simulink model "Sterowanie_StatkiemVIDI_2015"  (R2015b)
settings: Solver=FixedStepAuto  SolverMode=SingleTasking  StartTime=0.0  StopTime=10  FixedStep=0.001  MaxStep=0.01  MinStep=.009  RelTol=1e-2
settings Model: Creator=szymo  LastModifiedBy=szymo
settings SolverCC: AlgebraicLoopSolver=LineSearch
settings DataIOCC: LimitDataPoints=off  ReturnWorkspaceOutputs=on
settings DebuggingCC: AllowSymbolicDim=on  SFUnexpectedBacktrackingDiag=error  SFNoUnconditionalDefaultTransitionDiag=error
settings ModelReferenceCC: PropagateSignalLabelsOutOfModel=on
settings SFSimCC: SimUseLocalCustomCode=on
settings RTWCC: RTWUseLocalCustomCode=on
settings GRTTargetCC: TargetLangStandard=C99 (ISO)
settings ConfigComp: CovMetricSettings=dwe  CovHtmlReporting=off  CovSaveCumulativeToWorkspaceVar=off  CovSaveSingleToWorkspaceVar=off  CovModelRefEnable=Off  CovExternalEMLEnable=on

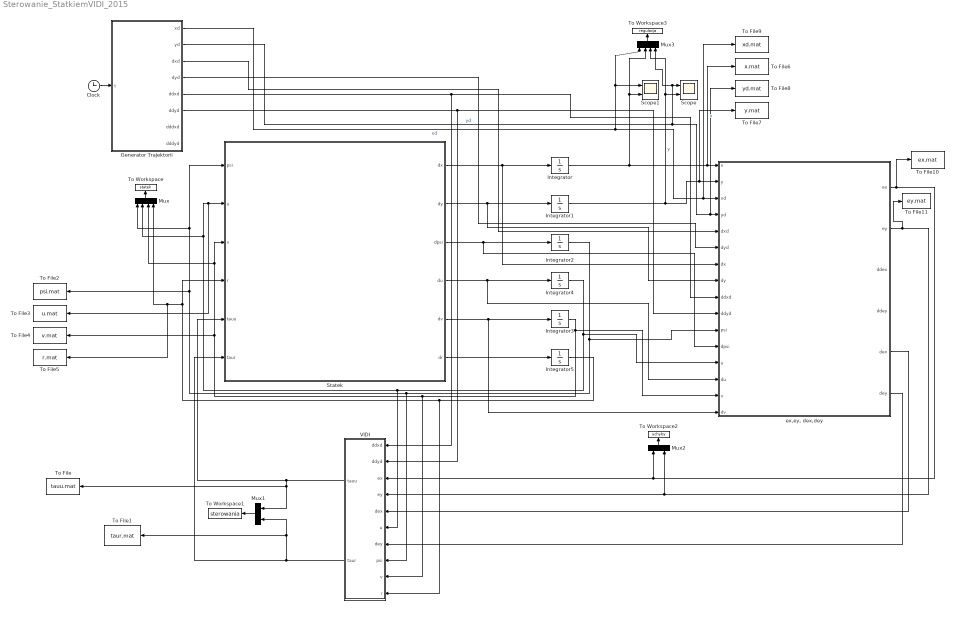
== system Sterowanie_StatkiemVIDI_2015 ==
  Clock : Clock
  Generator Trajektorii : MATLAB Function  TreatAsAtomicUnit=on
  Integrator : Integrator  InitialCondition=-0.01
  Integrator1 : Integrator  InitialCondition=1.01
  Integrator2 : Integrator  InitialCondition=0.01
  Integrator3 : Integrator  InitialCondition=0.1
  Integrator4 : Integrator  InitialCondition=0.1
  Integrator5 : Integrator  InitialCondition=0.1
  Mux : Mux
  Mux1 : Mux  Inputs=2
  Mux2 : Mux  Inputs=2
  Mux3 : Mux
  Scope : Scope  NumInputPorts=2
  Scope1 : Scope  NumInputPorts=2
  Statek : MATLAB Function  TreatAsAtomicUnit=on
  To File : ToFile  Filename=tauu.mat  SaveFormat=Timeseries
  To File1 : ToFile  Filename=taur.mat  SaveFormat=Timeseries
  To File10 : ToFile  Filename=ex.mat  SaveFormat=Timeseries
  To File11 : ToFile  Filename=ey.mat  SaveFormat=Timeseries
  To File2 : ToFile  Filename=psi.mat  SaveFormat=Timeseries
  To File3 : ToFile  Filename=u.mat  SaveFormat=Timeseries
  To File4 : ToFile  Filename=v.mat  SaveFormat=Timeseries
  To File5 : ToFile  Filename=r.mat  SaveFormat=Timeseries
  To File6 : ToFile  Filename=x.mat  SaveFormat=Timeseries
  To File7 : ToFile  Filename=y.mat  SaveFormat=Timeseries
  To File8 : ToFile  Filename=yd.mat  SaveFormat=Timeseries
  To File9 : ToFile  Filename=xd.mat  SaveFormat=Timeseries
  To Workspace : ToWorkspace  VariableName=statek  SaveFormat=Timeseries  SampleTime=-1
  To Workspace1 : ToWorkspace  VariableName=sterowania  SaveFormat=Timeseries  SampleTime=-1
  To Workspace2 : ToWorkspace  VariableName=uchyby  SaveFormat=Timeseries  SampleTime=-1
  To Workspace3 : ToWorkspace  VariableName=regulacja  SaveFormat=Timeseries  SampleTime=-1
  VIDI : Subsystem
  "ex,ey, dex,dey" : MATLAB Function  TreatAsAtomicUnit=on
  wires:
  Clock/1 -> Generator Trajektorii/1(t)
  Generator Trajektorii/1(xd) -> Scope1/1, Mux3/1, To File9/1, "ex,ey, dex,dey"/3(xd)  "xd"
  Statek/1(dx) -> "ex,ey, dex,dey"/7(dx), Integrator/1
  Statek/2(dy) -> "ex,ey, dex,dey"/8(dy), Integrator1/1
  Statek/3(dpsi) -> "ex,ey, dex,dey"/12(dpsi), Integrator2/1
  Statek/4(du) -> "ex,ey, dex,dey"/14(du), Integrator4/1
  Statek/5(dv) -> "ex,ey, dex,dey"/16(dv), Integrator3/1
  Statek/6(dr) -> Integrator5/1
  Integrator/1 -> Mux3/2, Scope1/2, To File6/1, "ex,ey, dex,dey"/1(x)  "x"
  Integrator1/1 -> Mux3/3, Scope/2, To File7/1, "ex,ey, dex,dey"/2(y)  "y"
  Generator Trajektorii/2(yd) -> Mux3/4, Scope/1, To File8/1, "ex,ey, dex,dey"/4(yd)  "yd"
  Generator Trajektorii/5(ddxd) -> "ex,ey, dex,dey"/9(ddxd), VIDI/1(ddxd)
  Generator Trajektorii/6(ddyd) -> VIDI/2(ddyd), "ex,ey, dex,dey"/10(ddyd)
  Integrator2/1 -> "ex,ey, dex,dey"/11(psi), Statek/1(psi), Mux/1, To File2/1, VIDI/8(psi)
  Integrator5/1 -> VIDI/10(r), To File5/1, Mux/4, Statek/4(r)
  Generator Trajektorii/3(dxd) -> "ex,ey, dex,dey"/5(dxd)
  Generator Trajektorii/4(dyd) -> "ex,ey, dex,dey"/6(dyd)
  Integrator4/1 -> "ex,ey, dex,dey"/13(u), Mux/2, To File3/1, Statek/2(u), VIDI/6(u)
  Integrator3/1 -> "ex,ey, dex,dey"/15(v), Statek/3(v), Mux/3, To File4/1, VIDI/9(v)
  "ex,ey, dex,dey"/1(ex) -> To File10/1, VIDI/3(ex), Mux2/1
  "ex,ey, dex,dey"/2(ey) -> To File11/1, Mux2/2, VIDI/4(ey)
  "ex,ey, dex,dey"/5(dex) -> VIDI/5(dex)
  "ex,ey, dex,dey"/6(dey) -> VIDI/7(dey)
  VIDI/1(tauu) -> To File/1, Mux1/1, Statek/5(tauu)
  VIDI/2(taur) -> To File1/1, Mux1/2, Statek/6(taur)
  Mux/1 -> To Workspace/1
  Mux1/1 -> To Workspace1/1
  Mux2/1 -> To Workspace2/1
  Mux3/1 -> To Workspace3/1

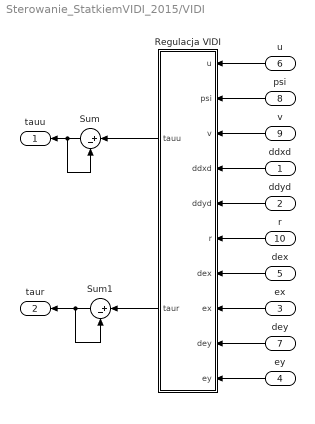
== system Sterowanie_StatkiemVIDI_2015/VIDI ==
  ddxd : Inport
  ddyd : Inport  Port=2
  ex : Inport  Port=3
  ey : Inport  Port=4
  dex : Inport  Port=5
  u : Inport  Port=6
  dey : Inport  Port=7
  psi : Inport  Port=8
  v : Inport  Port=9
  r : Inport  Port=10
  Regulacja VIDI : MATLAB Function  TreatAsAtomicUnit=on
  Sum : Sum  Inputs=|+-
  Sum1 : Sum  Inputs=|+-
  tauu : Outport
  taur : Outport  Port=2
  wires:
  ddxd/1 -> Regulacja VIDI/4(ddxd)
  Regulacja VIDI/2(taur) -> Sum1/1
  Sum/1 -> Sum/2, tauu/1
  ey/1 -> Regulacja VIDI/10(ey)
  Regulacja VIDI/1(tauu) -> Sum/1
  v/1 -> Regulacja VIDI/3(v)
  psi/1 -> Regulacja VIDI/2(psi)
  Sum1/1 -> Sum1/2, taur/1
  u/1 -> Regulacja VIDI/1(u)
  dey/1 -> Regulacja VIDI/9(dey)
  ddyd/1 -> Regulacja VIDI/5(ddyd)
  dex/1 -> Regulacja VIDI/7(dex)
  ex/1 -> Regulacja VIDI/8(ex)
  r/1 -> Regulacja VIDI/6(r)

== matlab function Sterowanie_StatkiemVIDI_2015/Generator Trajektorii ==
  data: t input; xd output; yd output; dxd output; dyd output; ddxd output; ddyd output; dddxd output; dddyd output
function [xd,yd,dxd,dyd,ddxd,ddyd,dddxd,dddyd] = fcn(t)

xd = sin(t);
yd = cos(t);
dxd=cos(t);
dyd=-sin(t);
ddxd = -sin(t);
ddyd = -cos(t);
dddxd = -cos(t);
dddyd = sin(t);

== matlab function Sterowanie_StatkiemVIDI_2015/Statek ==
  data: psi input size=1; u input size=1; v input size=1; dx output size=1; r input size=1; dy output size=1; dpsi output size=1; du output size=1; dv output size=1; dr output size=1; tauu input size=1; taur input size=1
function [dx,dy,dpsi,du,dv,dr] = fcn(psi,u,v,r,tauu,taur)
m11=1.956;
m22=2.405;
m33=0.043;
d11=2.436;
d22=12.992;
d33=0.0564;
dx = u*cos(psi)-v*sin(psi);
dy = u*sin(psi)+v*cos(psi);
dpsi = r;
du = (m22*v*r-d11*u+tauu)/m11;
dv = (-m11*u*r-d22*v)/m22;
dr = ((m11-m22)*u*v-d33*r+taur)/m33;

== matlab function Sterowanie_StatkiemVIDI_2015/ex,ey, dex,dey ==
  data: x input; y input; xd input; yd input; dxd input; dyd input; dx input; dy input; ddxd input; ddyd input; psi input; dpsi input; u input; du input; v input; dv input; ex output; ey output; ddex output; ddey output; dex output; dey output
function [ex,ey,ddex,ddey,dex,dey] = fcn(x,y,xd,yd,dxd,dyd,dx,dy,ddxd,ddyd,psi,dpsi,u,du,v,dv)

ex = x-xd;
ey = y-yd;
m11=1.956;
dex=dx-dxd;
dey=dy-dyd;
ddex = du*cos(psi)-u*dpsi*sin(psi)-dv*sin(psi)-v*dpsi*cos(psi)-ddxd;
ddey = du*sin(psi)+u*dpsi*cos(psi)+dv*cos(psi)-v*dpsi*sin(psi)-ddyd;

== matlab function Sterowanie_StatkiemVIDI_2015/VIDI/Regulacja VIDI ==
  data: u input; tauu output; psi input; v input; ddxd input; ddyd input; r input; dex input; ex input; dey input; ey input; taur output
function [tauu, taur] = fcn(u,psi,v,ddxd,ddyd,r,dex,ex,dey,ey)
k21=10; %pogorszyl
k22=10; %ten na 10, reszta na 1 daje dobrego x
k23=10; %pogorszyl
k24=10; %przyblizyl y ale nie tak szybko
k25=2;% blad symulacji
lambda=10;
m11=1.956;
m22=2.405;
m33=0.043;
d11=2.436;
d22=12.992;
d33=0.0564;

fr = ((m11-m22)*u*v-d33*r)/m33;
gr = 1/m33;

G2 = [cos(psi)/m11 m22*v*cos(psi)/m11+m11*u*sin(psi)/m22-u*sin(psi)-v*cos(psi); sin(psi)/m11 m22*v*sin(psi)/m11-m11*u*cos(psi)/m22+u*cos(psi)-v*sin(psi)];
F2 = [-d11*u*cos(psi)/m11+d22*v*sin(psi)*m22-ddxd; -d11*u*sin(psi)/m11-d22*v*cos(psi)/m22-ddyd];
wek = (G2)^(-1)*(-1*F2+[-k21*dex-k22*ex;-k23*dey-k24*ey]);
tauu = wek(1);
rd = wek(2);
taur = gr^(-1)*(lambda*(rd-r)-fr-k25*(rd-r));
